simulink model "leon_chen_TDPBehaviourSim2"  (R2020b)
settings: Solver=FixedStepDiscrete  StartTime=0.0  StopTime=inf  RelTol=1e-3  EnableMultiTasking=on
values from neighbouring files (symbols this model uses):
  angThresh = pi/16    (= 0.196349540849)    [GameParameters.m]
  attackerKickSpeed = 0.3    [GameParameters.m]
  AwayFormation1 = [9.5 4 pi ... (first row only)    [FormationPoses.m]    (also in GameParameters.m)
  ballThresh = playerRadius + 0.03    (= 0.11)    [GameParameters.m]
  distThresh = 0.1    [GameParameters.m]
  fieldCenter = [mean(fieldLimitsX) mean(fieldLimitsY)]    [GameParameters.m]
  fieldLimitsX = [1 10]    [GameParameters.m]
  fieldLimitsY = [1 7]    [GameParameters.m]
  goalPosts = [1  2.7 2 ... (first row only)    [GameParameters.m]
  HomeFormation1 = [1.5 4 0 ... (first row only)    [FormationPoses.m]    (also in GameParameters.m)
  maxSpeed = 0.1    [GameParameters.m]
  maxTurnSpeed = 0.05    [GameParameters.m]
  playerRadius = 0.08    [GameParameters.m]
  robotDetectorAngle = 0    [GameParameters.m]
  robotDetectorFOV = 4.15    [GameParameters.m]
  robotDetectorMaxHits = 7    [GameParameters.m]
  robotDetectorOffset = [0 0]    [GameParameters.m]
  robotDetectorRange = 10    [GameParameters.m]
  sampleTime = 0.5    [GameParameters.m]
undefined symbols (not defined in the file or in its folder): DiscIntNeverNeededParam
libraries: mobileRoboticsLib x28, soccerRobotLib x16
(part 2 of 2)

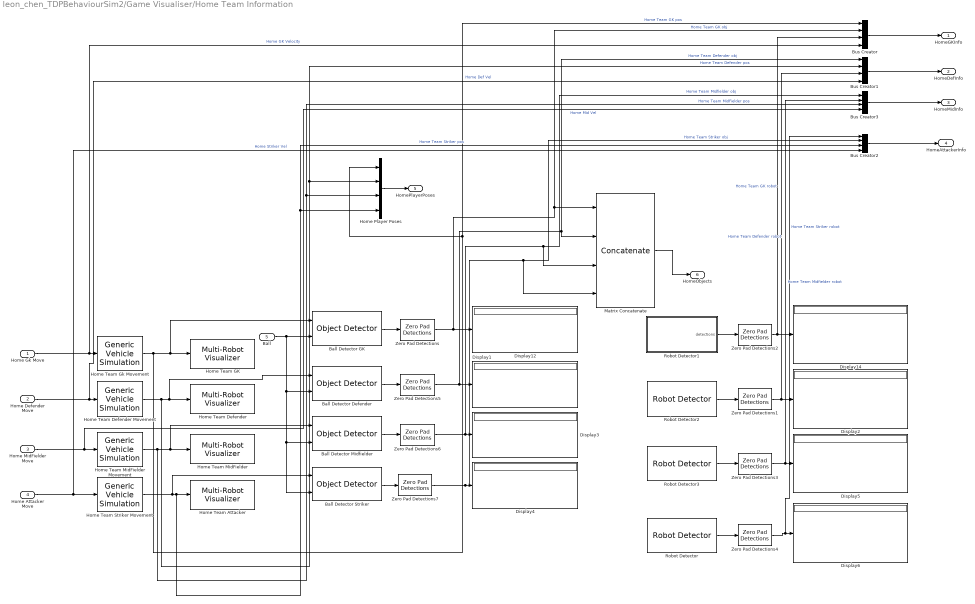
== system leon_chen_TDPBehaviourSim2/Game Visualiser/Home Team Information ==
  Home Gk Move : Inport
  Home Defender Move : Inport  Port=2
  Home MidFielder Move : Inport  Port=3
  Home Attacker Move : Inport  Port=4
  Ball : Inport  Port=5
  Ball Detector Defender : mobileRoboticsLib/Environments/Object Detector  mapName=map  sensorOffset=objDetectorOffset  sensorAngle=objDetectorAngle  fieldOfView=objDetectorFOV  maxRange=objDetectorRange  maxDetections=objDetectorMaxHits  sampleTime=0.1
      settings: SourceProductName=Mobile Robotics Simulation Toolbox
  Ball Detector GK : mobileRoboticsLib/Environments/Object Detector  mapName=map  sensorOffset=objDetectorOffset  sensorAngle=objDetectorAngle  fieldOfView=objDetectorFOV  maxRange=objDetectorRange  maxDetections=objDetectorMaxHits  sampleTime=0.1
      settings: SourceProductName=Mobile Robotics Simulation Toolbox
  Ball Detector Midfielder : mobileRoboticsLib/Environments/Object Detector  mapName=map  sensorOffset=objDetectorOffset  sensorAngle=objDetectorAngle  fieldOfView=objDetectorFOV  maxRange=objDetectorRange  maxDetections=objDetectorMaxHits  sampleTime=0.1
      settings: SourceProductName=Mobile Robotics Simulation Toolbox
  Ball Detector Striker : mobileRoboticsLib/Environments/Object Detector  mapName=map  sensorOffset=objDetectorOffset  sensorAngle=objDetectorAngle  fieldOfView=objDetectorFOV  maxRange=objDetectorRange  maxDetections=objDetectorMaxHits  sampleTime=0.1
      settings: SourceProductName=Mobile Robotics Simulation Toolbox
  Bus Creator{,1..3} (4 alike) : BusCreator  Inputs=4
  Display{1..6,12,14} (8 alike) : Display
  Home Player Poses : BusCreator  Inputs=4
  Home Team Attacker : mobileRoboticsLib/Environments/Multi-Robot Visualizer  idx=4  radius=playerRadius  robotColor=homeTeamColor  showTraj=on  hasLidar=off  sensorOffset=[0,0]  scanAngles=[-pi/4 0 pi/4]  maxNumScans=0  hasObjDetector=on  objDetectorOffset=objDetectorOffset  objDetectorAngle=objDetectorAngle  objDetectorFOV=objDetectorFOV  objDetectorMaxRange=objDetectorMaxHits  hasRobotDetector=on  robotDetectorOffset=robotDetectorOffset  robotDetectorAngle=robotDetectorAngle  robotDetectorFOV=robotDetectorFOV  robotDetectorMaxRange=robotDetectorRange  robotDetectorNumDetections=0
      settings: SourceProductName=Mobile Robotics Simulation Toolbox
  Home Team Defender : mobileRoboticsLib/Environments/Multi-Robot Visualizer  idx=2  radius=playerRadius  robotColor=homeTeamColor  showTraj=on  hasLidar=off  sensorOffset=[0,0]  scanAngles=[-pi/4 0 pi/4]  maxNumScans=0  hasObjDetector=on  objDetectorOffset=objDetectorOffset  objDetectorAngle=objDetectorAngle  objDetectorFOV=objDetectorFOV  objDetectorMaxRange=objDetectorMaxHits  hasRobotDetector=off  robotDetectorOffset=[0,0]  robotDetectorAngle=0  robotDetectorFOV=pi/3  robotDetectorMaxRange=5  robotDetectorNumDetections=0
      settings: SourceProductName=Mobile Robotics Simulation Toolbox
  Home Team Defender Movement : mobileRoboticsLib/Utilities/Generic Vehicle Simulation  initX=HomeFormation1(2,1)  initY=HomeFormation1(2,2)  initAngle=HomeFormation1(2,3)  Ts=0.05
      settings: SourceProductName=Mobile Robotics Simulation Toolbox
  Home Team GK : mobileRoboticsLib/Environments/Multi-Robot Visualizer  idx=1  radius=playerRadius  robotColor=homeGKColor  showTraj=on  hasLidar=off  sensorOffset=[0,0]  scanAngles=[-pi/4 0 pi/4]  maxNumScans=0  hasObjDetector=on  objDetectorOffset=objDetectorOffset  objDetectorAngle=objDetectorAngle  objDetectorFOV=objDetectorFOV  objDetectorMaxRange=objDetectorRange  hasRobotDetector=on  robotDetectorOffset=robotDetectorOffset  robotDetectorAngle=robotDetectorAngle  robotDetectorFOV=robotDetectorFOV  robotDetectorMaxRange=robotDetectorRange  robotDetectorNumDetections=0
      settings: SourceProductName=Mobile Robotics Simulation Toolbox
  Home Team Gk Movement : mobileRoboticsLib/Utilities/Generic Vehicle Simulation  initX=HomeFormation1(1,1)  initY=HomeFormation1(1,2)  initAngle=HomeFormation1(1,3)  Ts=0.05
      settings: SourceProductName=Mobile Robotics Simulation Toolbox
  Home Team MidFielder : mobileRoboticsLib/Environments/Multi-Robot Visualizer  idx=3  radius=playerRadius  robotColor=homeTeamColor  showTraj=on  hasLidar=off  sensorOffset=[0,0]  scanAngles=[-pi/4 0 pi/4]  maxNumScans=0  hasObjDetector=off  objDetectorOffset=[0,0]  objDetectorAngle=0  objDetectorFOV=pi/3  objDetectorMaxRange=5  hasRobotDetector=off  robotDetectorOffset=[0,0]  robotDetectorAngle=0  robotDetectorFOV=pi/3  robotDetectorMaxRange=5  robotDetectorNumDetections=0
      settings: SourceProductName=Mobile Robotics Simulation Toolbox
  Home Team MidFielder Movement : mobileRoboticsLib/Utilities/Generic Vehicle Simulation  initX=HomeFormation1(3,1)  initY=HomeFormation1(3,2)  initAngle=HomeFormation1(3,3)  Ts=0.05
      settings: SourceProductName=Mobile Robotics Simulation Toolbox
  Home Team Striker Movement : mobileRoboticsLib/Utilities/Generic Vehicle Simulation  initX=HomeFormation1(4,1)  initY=HomeFormation1(4,2)  initAngle=HomeFormation1(4,3)  Ts=0.05
      settings: SourceProductName=Mobile Robotics Simulation Toolbox
  Matrix Concatenate : Concatenate  NumInputs=4  Mode=Multidimensional array
  Robot Detector : mobileRoboticsLib/Environments/Robot Detector  mapName=map  robotIdx=4  sensorOffset=robotDetectorOffset  sensorAngle=robotDetectorAngle  sensorFOV=robotDetectorFOV  maxRange=robotDetectorRange  maxDetections=robotDetectorMaxHits  sampleTime=sampleTime
      settings: SourceProductName=Mobile Robotics Simulation Toolbox
  Robot Detector1 : Subsystem  AncestorBlock=mobileRoboticsLib/Environments/Robot Detector  mask(Robot Detector){mapName=map, robotIdx=1, sensorOffset=robotDetectorOffset, sensorAngle=robotDetectorAngle, sensorFOV=robotDetectorFOV, maxRange=robotDetectorRange, maxDetections=robotDetectorMaxHits, sampleTime=sampleTime}
      mask prompts: mapName "Map Name"; robotIdx "Robot Index"; sensorOffset "Sensor offset (x,y) [m]"; sensorAngle "Sensor angle [rad]"; sensorFOV "Sensor field of view [rad]"; maxRange "Maximum range [rad]"; maxDetections "Maximum number of detections"; sampleTime "Sample Time"
      mask help: Robot Detector Simulator
      mask init: same as leon_chen_TDPBehaviourSim2/Game Visualiser/Away Team Information/Robot Detector1
      mask Help: web('matlab: edit mrsDocRobotDetector')
      mask Callback mapName:
      | % Update the map in the Robot Detector system object inside the mask
      | mapName = get_param(gcb,'mapName');
      | blkName = [gcb '/Robot Detector'];
      | set_param(blkName,'mapName',mapName);
      mask Display:
      | idx = get_param(gcb,'robotIdx');
      | fprintf(['Robot ' idx '\n Detector'])
  Robot Detector2 : mobileRoboticsLib/Environments/Robot Detector  mapName=map  robotIdx=2  sensorOffset=robotDetectorOffset  sensorAngle=robotDetectorAngle  sensorFOV=robotDetectorFOV  maxRange=robotDetectorRange  maxDetections=robotDetectorMaxHits  sampleTime=sampleTime
      settings: SourceProductName=Mobile Robotics Simulation Toolbox
  Robot Detector3 : mobileRoboticsLib/Environments/Robot Detector  mapName=map  robotIdx=3  sensorOffset=robotDetectorOffset  sensorAngle=robotDetectorAngle  sensorFOV=robotDetectorFOV  maxRange=robotDetectorRange  maxDetections=robotDetectorMaxHits  sampleTime=sampleTime
      settings: SourceProductName=Mobile Robotics Simulation Toolbox
  Zero Pad Detections{,5..7} (4 alike) : soccerRobotLib/Soccer Robot Simulator/Zero Pad Detections  maxHits=objDetectorMaxHits
  Zero Pad Detections{1..4} (4 alike) : soccerRobotLib/Soccer Robot Simulator/Zero Pad Detections  maxHits=robotDetectorMaxHits
  HomeGKInfo : Outport
  HomeDefInfo : Outport  Port=2
  HomeMidInfo : Outport  Port=3
  HomeAttackerInfo : Outport  Port=4
  HomePlayerPoses : Outport  Port=5
  HomeObjects : Outport  Port=6
  wires:
  Home Gk Move/1 -> Bus Creator/4, Home Team Gk Movement/1  "Home GK Velocity"
  Home Team Striker Movement/1 -> Bus Creator2/3, Home Player Poses/4, Home Team Attacker/1, Ball Detector Striker/1  "Home Team Striker pos"
  Home Attacker Move/1 -> Home Team Striker Movement/1, Bus Creator2/4  "Home Striker Vel"
  Home Defender Move/1 -> Bus Creator1/4, Home Team Defender Movement/1  "Home Def Vel"
  Home Team Gk Movement/1 -> Ball Detector GK/1, Home Team GK/1, Bus Creator/1, Home Player Poses/1  "Home Team GK pos"
  Home Team Defender Movement/1 -> Bus Creator1/2, Home Player Poses/2, Ball Detector Defender/1, Home Team Defender/1  "Home Team Defender pos"
  Home Team MidFielder Movement/1 -> Bus Creator3/3, Home Player Poses/3, Ball Detector Midfielder/1, Home Team MidFielder/1  "Home Team MidFielder pos"
  Home MidFielder Move/1 -> Bus Creator3/4, Home Team MidFielder Movement/1  "Home Mid Vel"
  Ball/1 -> Ball Detector Striker/2, Ball Detector Midfielder/2, Ball Detector Defender/2, Ball Detector GK/2
  Ball Detector GK/1 -> Zero Pad Detections/1
  Ball Detector Midfielder/1 -> Zero Pad Detections6/1
  Ball Detector Defender/1 -> Zero Pad Detections5/1
  Ball Detector Striker/1 -> Zero Pad Detections7/1
  Robot Detector1/1(detections) -> Zero Pad Detections2/1
  Robot Detector3/1 -> Zero Pad Detections3/1
  Robot Detector/1 -> Zero Pad Detections4/1
  Zero Pad Detections/1 -> Matrix Concatenate/1, Bus Creator/2, Display12/1  "Home Team GK obj"
  Zero Pad Detections2/1 -> Display14/1, Bus Creator/3  "Home Team GK robot"
  Zero Pad Detections1/1 -> Display2/1, Bus Creator1/3  "Home Team Defender robot"
  Robot Detector2/1 -> Zero Pad Detections1/1
  Zero Pad Detections3/1 -> Bus Creator3/2, Display5/1  "Home Team Midfielder robot"
  Zero Pad Detections4/1 -> Bus Creator2/1, Display6/1  "Home Team Striker robot"
  Zero Pad Detections5/1 -> Display1/1, Matrix Concatenate/2, Bus Creator1/1  "Home Team Defender obj"
  Zero Pad Detections6/1 -> Matrix Concatenate/3, Bus Creator3/1, Display3/1  "Home Team Midfielder obj"
  Zero Pad Detections7/1 -> Display4/1, Matrix Concatenate/4, Bus Creator2/2  "Home Team Striker obj"
  Home Player Poses/1 -> HomePlayerPoses/1
  Bus Creator/1 -> HomeGKInfo/1
  Bus Creator1/1 -> HomeDefInfo/1
  Bus Creator3/1 -> HomeMidInfo/1
  Bus Creator2/1 -> HomeAttackerInfo/1
  Matrix Concatenate/1 -> HomeObjects/1

== system leon_chen_TDPBehaviourSim2/Game Visualiser/Subsystem ==
  In5 : Inport
  Constant1 : Constant  Value=goalPosts
  Object Matrix Creator : MATLAB Function  TreatAsAtomicUnit=on
  objectPositions : Outport
  wires:
  Constant1/1 -> Object Matrix Creator/2(goalPosts)
  In5/1 -> Object Matrix Creator/1(BallPos)
  Object Matrix Creator/1(objectPositions) -> objectPositions/1

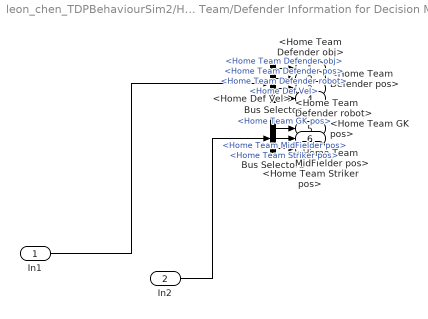
== system leon_chen_TDPBehaviourSim2/Home Team/Defender Information for Decision Making  ==
  In1 : Inport
  In2 : Inport  Port=2
  Bus Selector : BusSelector  OutputSignals=Home Team Defender obj,Home Team Defender pos,Home Team Defender robot,Home Def Vel
  Bus Selector1 : BusSelector  OutputSignals=Home Team GK pos,Home Team MidFielder pos,Home Team Striker pos
  <Home Team Defender obj> : Outport
  <Home Team Defender pos> : Outport  Port=2
  <Home Team Defender robot> : Outport  Port=3
  <Home Def Vel> : Outport  Port=4
  <Home Team GK pos> : Outport  Port=5
  <Home Team MidFielder pos> : Outport  Port=6
  <Home Team Striker pos> : Outport  Port=7
  wires:
  In1/1 -> Bus Selector/1
  In2/1 -> Bus Selector1/1
  Bus Selector1/2 -> <Home Team MidFielder pos>/1  "<Home Team MidFielder pos>"
  Bus Selector/3 -> <Home Team Defender robot>/1  "<Home Team Defender robot>"
  Bus Selector1/1 -> <Home Team GK pos>/1  "<Home Team GK pos>"
  Bus Selector1/3 -> <Home Team Striker pos>/1  "<Home Team Striker pos>"
  Bus Selector/4 -> <Home Def Vel>/1  "<Home Def Vel>"
  Bus Selector/1 -> <Home Team Defender obj>/1  "<Home Team Defender obj>"
  Bus Selector/2 -> <Home Team Defender pos>/1  "<Home Team Defender pos>"

== system leon_chen_TDPBehaviourSim2/Home Team/GK Information for Decision Making ==
  In1 : Inport
  In2 : Inport  Port=2
  Personal Information : BusSelector  OutputSignals=Home Team GK pos,Home Team GK obj,Home Team GK robot,Home GK Velocity
  TeamMatePositions : BusSelector  OutputSignals=Home Team Defender pos,Home Team MidFielder pos,Home Team Striker pos
  <Home Team GK pos> : Outport
  <Home Team GK obj> : Outport  Port=2
  <Home Team GK robot> : Outport  Port=3
  <Home GK Velocity> : Outport  Port=4
  <Home Team Defender pos> : Outport  Port=5
  <Home Team MidFielder pos> : Outport  Port=6
  <Home Team Striker pos> : Outport  Port=7
  wires:
  Personal Information/2 -> <Home Team GK obj>/1  "<Home Team GK obj>"
  Personal Information/4 -> <Home GK Velocity>/1  "<Home GK Velocity>"
  TeamMatePositions/3 -> <Home Team Striker pos>/1  "<Home Team Striker pos>"
  In1/1 -> Personal Information/1
  In2/1 -> TeamMatePositions/1
  Personal Information/1 -> <Home Team GK pos>/1  "<Home Team GK pos>"
  TeamMatePositions/1 -> <Home Team Defender pos>/1  "<Home Team Defender pos>"
  Personal Information/3 -> <Home Team GK robot>/1  "<Home Team GK robot>"
  TeamMatePositions/2 -> <Home Team MidFielder pos>/1  "<Home Team MidFielder pos>"

== system leon_chen_TDPBehaviourSim2/Home Team/MidFielder Information For Decision Making ==
  In1 : Inport
  In2 : Inport  Port=2
  Bus Selector : BusSelector  OutputSignals=Home Team Midfielder obj,Home Team Midfielder robot,Home Team MidFielder pos,Home Mid Vel
  Bus Selector1 : BusSelector  OutputSignals=Home Team Striker pos,Home Team Defender pos,Home Team GK pos
  <Home Team Midfielder obj> : Outport
  <Home Team Midfielder robot> : Outport  Port=2
  <Home Team MidFielder pos> : Outport  Port=3
  <Home Mid Vel> : Outport  Port=4
  <Home Team Striker pos> : Outport  Port=5
  <Home Team Defender pos> : Outport  Port=6
  <Home Team GK pos> : Outport  Port=7
  wires:
  Bus Selector1/3 -> <Home Team GK pos>/1  "<Home Team GK pos>"
  Bus Selector1/1 -> <Home Team Striker pos>/1  "<Home Team Striker pos>"
  Bus Selector/1 -> <Home Team Midfielder obj>/1  "<Home Team Midfielder obj>"
  In2/1 -> Bus Selector/1
  In1/1 -> Bus Selector1/1
  Bus Selector1/2 -> <Home Team Defender pos>/1  "<Home Team Defender pos>"
  Bus Selector/2 -> <Home Team Midfielder robot>/1  "<Home Team Midfielder robot>"
  Bus Selector/3 -> <Home Team MidFielder pos>/1  "<Home Team MidFielder pos>"
  Bus Selector/4 -> <Home Mid Vel>/1  "<Home Mid Vel>"

== system leon_chen_TDPBehaviourSim2/Home Team/Striker Information fot Decision Making ==
  In1 : Inport
  In2 : Inport  Port=2
  Bus Selector : BusSelector  OutputSignals=Home Team Striker robot,Home Team Striker obj,Home Team Striker pos,Home Striker Vel
  Bus Selector1 : BusSelector  OutputSignals=Home Team GK pos,Home Team Defender pos,Home Team MidFielder pos
  <Home Team Striker robot> : Outport
  <Home Team Striker obj> : Outport  Port=2
  <Home Team Striker pos> : Outport  Port=3
  <Home Striker Vel> : Outport  Port=4
  <Home Team GK pos> : Outport  Port=5
  <Home Team Defender pos> : Outport  Port=6
  <Home Team MidFielder pos> : Outport  Port=7
  wires:
  Bus Selector1/1 -> <Home Team GK pos>/1  "<Home Team GK pos>"
  In1/1 -> Bus Selector/1
  In2/1 -> Bus Selector1/1
  Bus Selector/1 -> <Home Team Striker robot>/1  "<Home Team Striker robot>"
  Bus Selector/4 -> <Home Striker Vel>/1  "<Home Striker Vel>"
  Bus Selector/2 -> <Home Team Striker obj>/1  "<Home Team Striker obj>"
  Bus Selector/3 -> <Home Team Striker pos>/1  "<Home Team Striker pos>"
  Bus Selector1/3 -> <Home Team MidFielder pos>/1  "<Home Team MidFielder pos>"
  Bus Selector1/2 -> <Home Team Defender pos>/1  "<Home Team Defender pos>"

== system leon_chen_TDPBehaviourSim2/Game Visualiser/Away Team Information/Robot Detector1 ==
  Poses : Subsystem
  Robot Detector : MATLABSystem  System=RobotDetector  mapName=map  robotIdx=robotIdx  sensorOffset=sensorOffset  sensorAngle=sensorAngle  fieldOfView=sensorFOV  maxRange=maxRange  maxDetections=maxDetections  sampleTime=sampleTime
      mask Type: RobotDetector
      mask Display:
      | disp(['Robot 5' char(10) 'Detector']);
      | port_label('output',1,'detections');
  detections : Outport  VectorParamsAs1DForOutWhenUnconnected=off
  wires:
  Poses/1(poses) -> Robot Detector/1
  Robot Detector/1 -> detections/1

== system leon_chen_TDPBehaviourSim2/Game Visualiser/Away Team Information/Robot Detector2 ==
  Poses : Subsystem
  Robot Detector : MATLABSystem  System=RobotDetector  mapName=map  robotIdx=robotIdx  sensorOffset=sensorOffset  sensorAngle=sensorAngle  fieldOfView=sensorFOV  maxRange=maxRange  maxDetections=maxDetections  sampleTime=sampleTime
      mask Type: RobotDetector
      mask Display:
      | disp(['Robot 8' char(10) 'Detector']);
      | port_label('output',1,'detections');
  detections : Outport  VectorParamsAs1DForOutWhenUnconnected=off
  wires:
  Poses/1(poses) -> Robot Detector/1
  Robot Detector/1 -> detections/1

== system leon_chen_TDPBehaviourSim2/Game Visualiser/Away Team Information/Robot Detector3 ==
  Poses : Subsystem
  Robot Detector : MATLABSystem  System=RobotDetector  mapName=map  robotIdx=robotIdx  sensorOffset=sensorOffset  sensorAngle=sensorAngle  fieldOfView=sensorFOV  maxRange=maxRange  maxDetections=maxDetections  sampleTime=sampleTime
      mask Type: RobotDetector
      mask Display:
      | disp(['Robot 7' char(10) 'Detector']);
      | port_label('output',1,'detections');
  detections : Outport  VectorParamsAs1DForOutWhenUnconnected=off
  wires:
  Poses/1(poses) -> Robot Detector/1
  Robot Detector/1 -> detections/1

== system leon_chen_TDPBehaviourSim2/Game Visualiser/Away Team Information/Robot Detector4 ==
  Poses : Subsystem
  Robot Detector : MATLABSystem  System=RobotDetector  mapName=map  robotIdx=robotIdx  sensorOffset=sensorOffset  sensorAngle=sensorAngle  fieldOfView=sensorFOV  maxRange=maxRange  maxDetections=maxDetections  sampleTime=sampleTime
      mask Type: RobotDetector
      mask Display:
      | disp(['Robot 6' char(10) 'Detector']);
      | port_label('output',1,'detections');
  detections : Outport  VectorParamsAs1DForOutWhenUnconnected=off
  wires:
  Poses/1(poses) -> Robot Detector/1
  Robot Detector/1 -> detections/1

== system leon_chen_TDPBehaviourSim2/Game Visualiser/Home Team Information/Robot Detector1 ==
  Poses : Subsystem
  Robot Detector : MATLABSystem  System=RobotDetector  mapName=map  robotIdx=robotIdx  sensorOffset=sensorOffset  sensorAngle=sensorAngle  fieldOfView=sensorFOV  maxRange=maxRange  maxDetections=maxDetections  sampleTime=sampleTime
      mask Type: RobotDetector
      mask Display:
      | disp(['Robot 1' char(10) 'Detector']);
      | port_label('output',1,'detections');
  detections : Outport  VectorParamsAs1DForOutWhenUnconnected=off
  wires:
  Poses/1(poses) -> Robot Detector/1
  Robot Detector/1 -> detections/1

== system leon_chen_TDPBehaviourSim2/Game Visualiser/Away Team Information/Robot Detector1/Poses ==
  Vector Concatenate : Concatenate  NumInputs=8  Mode=Multidimensional array  ConcatenateDimension=2
  poses : Outport
  wires:
  Vector Concatenate/1 -> poses/1
  [slMultiRobotEnv_Pose_1] -> Vector Concatenate/1
  [slMultiRobotEnv_Pose_2] -> Vector Concatenate/2
  [slMultiRobotEnv_Pose_3] -> Vector Concatenate/3
  [slMultiRobotEnv_Pose_4] -> Vector Concatenate/4
  [slMultiRobotEnv_Pose_5] -> Vector Concatenate/5
  [slMultiRobotEnv_Pose_6] -> Vector Concatenate/6
  [slMultiRobotEnv_Pose_7] -> Vector Concatenate/7
  [slMultiRobotEnv_Pose_8] -> Vector Concatenate/8

== system leon_chen_TDPBehaviourSim2/Game Visualiser/Away Team Information/Robot Detector2/Poses ==
  Vector Concatenate : Concatenate  NumInputs=8  Mode=Multidimensional array  ConcatenateDimension=2
  poses : Outport
  wires:
  Vector Concatenate/1 -> poses/1
  [slMultiRobotEnv_Pose_1] -> Vector Concatenate/1
  [slMultiRobotEnv_Pose_2] -> Vector Concatenate/2
  [slMultiRobotEnv_Pose_3] -> Vector Concatenate/3
  [slMultiRobotEnv_Pose_4] -> Vector Concatenate/4
  [slMultiRobotEnv_Pose_5] -> Vector Concatenate/5
  [slMultiRobotEnv_Pose_6] -> Vector Concatenate/6
  [slMultiRobotEnv_Pose_7] -> Vector Concatenate/7
  [slMultiRobotEnv_Pose_8] -> Vector Concatenate/8

== system leon_chen_TDPBehaviourSim2/Game Visualiser/Away Team Information/Robot Detector3/Poses ==
  Vector Concatenate : Concatenate  NumInputs=8  Mode=Multidimensional array  ConcatenateDimension=2
  poses : Outport
  wires:
  Vector Concatenate/1 -> poses/1
  [slMultiRobotEnv_Pose_1] -> Vector Concatenate/1
  [slMultiRobotEnv_Pose_2] -> Vector Concatenate/2
  [slMultiRobotEnv_Pose_3] -> Vector Concatenate/3
  [slMultiRobotEnv_Pose_4] -> Vector Concatenate/4
  [slMultiRobotEnv_Pose_5] -> Vector Concatenate/5
  [slMultiRobotEnv_Pose_6] -> Vector Concatenate/6
  [slMultiRobotEnv_Pose_7] -> Vector Concatenate/7
  [slMultiRobotEnv_Pose_8] -> Vector Concatenate/8

== system leon_chen_TDPBehaviourSim2/Game Visualiser/Away Team Information/Robot Detector4/Poses ==
  Vector Concatenate : Concatenate  NumInputs=8  Mode=Multidimensional array  ConcatenateDimension=2
  poses : Outport
  wires:
  Vector Concatenate/1 -> poses/1
  [slMultiRobotEnv_Pose_1] -> Vector Concatenate/1
  [slMultiRobotEnv_Pose_2] -> Vector Concatenate/2
  [slMultiRobotEnv_Pose_3] -> Vector Concatenate/3
  [slMultiRobotEnv_Pose_4] -> Vector Concatenate/4
  [slMultiRobotEnv_Pose_5] -> Vector Concatenate/5
  [slMultiRobotEnv_Pose_6] -> Vector Concatenate/6
  [slMultiRobotEnv_Pose_7] -> Vector Concatenate/7
  [slMultiRobotEnv_Pose_8] -> Vector Concatenate/8

== system leon_chen_TDPBehaviourSim2/Game Visualiser/Home Team Information/Robot Detector1/Poses ==
  Vector Concatenate : Concatenate  NumInputs=8  Mode=Multidimensional array  ConcatenateDimension=2
  poses : Outport
  wires:
  Vector Concatenate/1 -> poses/1
  [slMultiRobotEnv_Pose_1] -> Vector Concatenate/1
  [slMultiRobotEnv_Pose_2] -> Vector Concatenate/2
  [slMultiRobotEnv_Pose_3] -> Vector Concatenate/3
  [slMultiRobotEnv_Pose_4] -> Vector Concatenate/4
  [slMultiRobotEnv_Pose_5] -> Vector Concatenate/5
  [slMultiRobotEnv_Pose_6] -> Vector Concatenate/6
  [slMultiRobotEnv_Pose_7] -> Vector Concatenate/7
  [slMultiRobotEnv_Pose_8] -> Vector Concatenate/8

== stateflow chart leon_chen_TDPBehaviourSim2/GamteState ==
  state BallNotHeld
    en,du:
    possession=[false,0];
    [x,y]=findholder(HomeObjects,AwayObjects);
  state BallHeld
    en,du:
    possession=[x,y];
    [x,y]=findholder(HomeObjects,AwayObjects);
  (default) -> BallNotHeld
  BallNotHeld -> BallHeld : [x==true]
  BallHeld -> BallNotHeld : [x==false]
  data: home function_input; holded function_output; indexholder function_output; away function_input; HomeObjects input; y local; x local; z local; possession output; AwayObjects input
  function [holded,indexholder]=findholder(home,away):
    | function [holded,indexholder]=findholder(home,away)
    | holded=false;
    | indexholder=0;
    | %% This function returns if ball is holded or not and the player's index if holded
    | for j=1:20
    |     %%
    |     % Test for Home Team
    |     %%
    |     if home(j,1)<=0.2 && home(j,1)>0 && home(j,2)<0.05 && home(j,2)>-0.05 && home(j,3)==1 %%&& 
    |         holded=true;
    |         if j==1
    |             indexholder=1;
    |         elseif j==6
    |             indexholder=2;
    |         elseif j==11
    |             indexholder=3;
    |         elseif j==16
    |             indexholder=4;
    |             
    |         end
    |         
    |         
    |     end
    |     %%
    |     % Test for Away Team
    |     %%
    |     if away(j,1)<=0.2 && away(j,1)>0 && away(j,2)<0.05 && away(j,2)>-0.05 && away(j,3)==1 %% && away(j,2)==0
    |         holded=true;
    |         if j==1
    |             indexholder=8;
    |         elseif j==6
    |             indexholder=7;
    |         elseif j==11
    |             indexholder=6;
    |         elseif j==16
    |             indexholder=5;
    |             
    |         end
    |         
    |         
    |     end
    | end

== matlab function leon_chen_TDPBehaviourSim2/Game Visualiser/Plot Soccer Field ==
function plotSoccerField
% Plots the soccer field once the figure window for the environment has
% been initialized

coder.extrinsic('evalin');
persistent hasPlotted
if isempty(hasPlotted)
    evalin('base','plotSoccerField');
    hasPlotted = true;
end

== matlab function leon_chen_TDPBehaviourSim2/Game Visualiser/Subsystem/Object Matrix Creator ==
  data: BallPos input; objectPositions output; goalPosts input
function objectPositions = SetPositions(BallPos,goalPosts)

objectPositions =[BallPos(1) BallPos(2) 1;goalPosts];

== stateflow chart leon_chen_TDPBehaviourSim2/Home Team/Chart ==
  state vel = trackDetection(dist,ang) [function]
    note: Uses range and bearing to track an object
    (default) -> (junction 79) : {
        | vel = [0;0;0];
        | }
    (junction 79) -> (junction 78) [order 1] : % Turn in place
        | % if no detection
        | [dist < 0]
    (junction 78) -> (junction 88) : {vel(3) = 1;}
    (junction 79) -> (junction 80) [order 2]
    (junction 80) -> (junction 81) [order 1] : % Forward speed
        | [dist > distThresh]
    (junction 81) -> (junction 83) : {vel(1) = maxSpeed;}
    (junction 80) -> (junction 82) [order 2]
    (junction 83) -> (junction 82)
    (junction 82) -> (junction 84)
    (junction 84) -> (junction 85) [order 1] : % Turning speed
        | [ang > angThresh]
    (junction 85) -> (junction 91) : {vel(3) = maxTurnSpeed;}
    (junction 84) -> (junction 86) [order 2]
    (junction 86) -> (junction 87) [order 1] : [ang < -angThresh]
    (junction 86) -> (junction 89) [order 2]
    (junction 87) -> (junction 90) : {vel(3) = -1;}
    (junction 88) -> (junction 89)
    (junction 90) -> (junction 89)
    (junction 91) -> (junction 90)
  state Information
    en,du:
    [objSeen,objDist,objAng] = detectObj(objects,1);
    [plSeen,plDist,plAng] = nearestHomePlayer(players);
    position;
    nextVelocity = trackDetection(objDist,objAng);
  state [vel,done] = turnToPoint(goal) [function]
    note: Tracks a position. Once reached, the robot will turn in place until a reference angle is met.
    (default) -> (junction 117) : % Turn in place until the angular reference is met
        | {
        | done = false;
        | vel = [0;0;0];
        | [goalDist,goalAng] = calcBearing(goal(1:2));
        | }
    (junction 117) -> (junction 118) [order 1] : [goalAng > angThresh]
    (junction 117) -> (junction 119) [order 2]
    (junction 118) -> (junction 123) : {vel(3) = 1;}
    (junction 119) -> (junction 120) [order 1] : [goalAng < -angThresh]
    (junction 119) -> (junction 121) [order 2] : {done = true;}
    (junction 120) -> (junction 122) : {vel(3) = -1;}
    (junction 122) -> (junction 121)
    (junction 123) -> (junction 122)
  state [vel,done] = goToPose(goal) [function]
    note: Tracks a position. Once reached, the robot will turn in place until a reference angle is met.
    (default) -> (junction 138) : {
        | vel = [0;0;0];
        | [goalDist,goalAng] = calcBearing(goal(1:2));
        | trackAng = angdiff(position(3),goal(3));
        | }
    (junction 138) -> (junction 139) [order 1] : % Track the position if outside the distance threshold
        | [goalDist > distThresh]
    (junction 138) -> (junction 140) [order 2] : % Else, turn in place until the angular reference is met
    (junction 139) -> (junction 147) : {vel = trackDetection(goalDist,goalAng);}
    (junction 140) -> (junction 141) [order 1] : [trackAng > angThresh]
    (junction 140) -> (junction 142) [order 2]
    (junction 141) -> (junction 146) : {vel(3) = 1;}
    (junction 142) -> (junction 143) [order 1] : [trackAng < -angThresh]
    (junction 142) -> (junction 144) [order 2]
    (junction 143) -> (junction 145) : {vel(3) = -1;}
    (junction 145) -> (junction 144)
    (junction 146) -> (junction 145)
    (junction 147) -> (junction 146)
    (junction 144) -> (junction 148) : {done = (goalDist <= distThresh) && (abs(trackAng) <= angThresh);}
  state [dist,ang] = calcBearing(goal) [function]
    (default) -> (junction 168) : % Calculate distance and angle to location
        | {
        | err = goal(1:2) - [position(1) position(2)];
        | dist = norm(err);
        | ang = angdiff(position(3),atan2(err(2),err(1)));
        | }
  state GotoGoal
    en,du:
    [objSeen,objDist,objAng] = detectObj(objects,4);
    nextVelocity = trackDetection(objDist,objAng);
  (default) -> Information
  Information -> GotoGoal : [objDist<0.2 && objDist~=-1 ]
  data: dist function_input; ang function_input; vel function_output; goal function_input; vel function_output; done function_output; vel function_output; done function_output; goal function_input; goal function_input; dist function_output; ang function_output; position input; velocity input; nextVelocity output =[0;0;0]; players input; teammates input; objects input; y local; z local; objDist local; objAng local; objSeen local; plDist local; plSeen local; plAng local; distThresh parameter; angThresh parameter; maxSpeed parameter; maxTurnSpeed parameter

== stateflow chart leon_chen_TDPBehaviourSim2/Home Team/Chart1 ==
  state Information
    en,du:
    position;
    nextVelocity = [velocity(1) velocity(2) velocity(3)]
    teammates;
  (default) -> Information
  data: position input; velocity input; nextVelocity output =[0,0,0]; players input; teammates input; objects input

== stateflow chart leon_chen_TDPBehaviourSim2/Home Team/Chart2 ==
  state Information
    en,du:
    position;
    nextVelocity = [velocity(1)  velocity(2) velocity(3)]
    teammates;
    players;
    objects;
  (default) -> Information
  data: velocity input; nextVelocity output =[0,0,0]; players input; teammates input; objects input; position input

== stateflow chart leon_chen_TDPBehaviourSim2/Away Team/Chart ==
  state Information
    en,du:
    position;
    players;
    objects
    nextVelocity = [velocity(1) velocity(2) velocity(3)]
    teammates;
  (default) -> Information
  data: position input; velocity input; nextVelocity output =[0,0,0]; players input; teammates input; objects input

== stateflow chart leon_chen_TDPBehaviourSim2/Away Team/Chart1 ==
  state Information
    en,du:
    position;
    nextVelocity = [velocity(1) velocity(2) velocity(3)]
    teammates;
    players;
    objects;
  (default) -> Information
  data: position input; velocity input; nextVelocity output =[0,0,0]; players input; teammates input; objects input

== stateflow chart leon_chen_TDPBehaviourSim2/Away Team/Chart2 ==
  state Information
    en,du:
    position;
    nextVelocity = [velocity(1) velocity(2) velocity(3)]
    teammates;
    players;
    objects
  (default) -> Information
  data: position input; velocity input; nextVelocity output =[0,0,0]; players input; teammates input; objects input

== stateflow chart leon_chen_TDPBehaviourSim2/Away Team/Chart3 ==
  state Information
    en,du:
    position;
    nextVelocity = [velocity(1) velocity(2) velocity(3)]
    teammates;
    objects;
    players;
  (default) -> Information
  data: position input; velocity input; nextVelocity output =[0,0,0]; players input; teammates input; objects input

== stateflow chart leon_chen_TDPBehaviourSim2/Chart1 ==
  state rIdx = findPossession [function] [commented out]
    (default) -> (junction 72) [commented out]
    (junction 72) -> (junction 73) [commented out] : % If the robot that previously possessed the ball is still holding it, keep the same index
        | [(gameState.possession > 0) && ...
        | (commands(gameState.possession).action == RobotAction.HoldBall)]
    (junction 72) -> (junction 74) [commented out] : % Else, find another valid robot holder
        | {rIdx = findNearestHoldingRobot;}
    (junction 73) -> (junction 75) [commented out] : {rIdx = gameState.possession;}
    (junction 75) -> (junction 74) [commented out]
  state state = getGameState [function]
    note: Returns the game state depending on the position of the ball on the field
    (default) -> (junction 52)
    (junction 52) -> (junction 53) [order 1] : [ballPose(1) <= fieldLimitsX(1) || ballPose(1) >= fieldLimitsX(2) || ...
        |  ballPose(2) <= fieldLimitsY(1) || ballPose(2) >= fieldLimitsY(2)]
    (junction 52) -> (junction 56) [order 2] : {state = gameSituation.InPlay;}
    (junction 53) -> (junction 54)
    (junction 54) -> (junction 55) [order 1] : [ballPose(2)<=goalPosts(1,2) && ...
        | ballPose(2) >= goalPosts(2,2)]
    (junction 54) -> (junction 57) [order 2] : {state = gameSituation.OutOfPlay;}
    (junction 55) -> (junction 58) : {state = gameSituation.GoalScored;}
    (junction 57) -> (junction 56)
    (junction 58) -> (junction 57)
  state BallDynamics [parallel]
    en:
    coder.extrinsic('randn'); % Lets us use MATLAB's interpreted RNG
    setBallState(fieldCenter,0,0);
    gamestate.state = getGameState;
    settings: executionOrder=1
    state InBounds
      en, du:
      state BallFree
      (default) -> BallFree
    state BallHeld
      en,du:
      ballPose = [robo_pos(3*hold_idx(2)-2) robo_pos(3*hold_idx(2)-1)] + ...
      (playerRadius+ballThresh)*[cos(robo_pos(3*hold_idx(2))) sin(robo_pos(3*hold_idx(2)))];
    (default) -> InBounds
    InBounds -> BallHeld : [hold_idx(1)~=0]
    BallHeld -> InBounds : [hold_idx(1)== 0]
  state setBallState(pos,vel,theta) [function]
  state Para [parallel] [commented out]
    en,du:
    ballDist = norm(robo_pos(1:2)-ballPose');
  data: nearIdx function_output size=1; rIdx function_output; state function_output; sf_internal_action_state_placeholder_data local double size=1 =0; pos function_input double size=[1 2]; vel function_input double size=1; theta function_input double size=1; ballPose output; gamestate local Bus: gameSituationBus; attackerKickSpeed parameter; ballThresh parameter; ballDist local; playerRadius parameter double; fieldLimitsX parameter; fieldLimitsY parameter; goalPosts parameter; fieldCenter parameter; robo_pos input; hold_idx input
  function nearIdx = findNearestHoldingRobot:
    | function nearIdx = findNearestHoldingRobot
    | % Finds possession based on the commands to all the robots 
    | % and their distances to the ball
    | 
    | [~,inds] = sort(ballDists);
    | rIdx = 0;
    | for idx = 1:numRobots
    |     if (commands(inds(idx)).action == RobotAction.HoldBall) && ....
    |        (ballDists(inds(idx)) <= ballThresh)
    |         rIdx = inds(idx);
    |         return;
    |     end
    | end
    | 
    | end

== stateflow chart leon_chen_TDPBehaviourSim2/Home Team/Chart3 ==
  state Information
    en,du:
    position;
    nextVelocity = [velocity(1) velocity(2) velocity(3)]
    teammates;
    players;
    objects;
  (default) -> Information
  data: position input; velocity input; nextVelocity output =[0,0,0]; players input; teammates input; objects input
